simulink subsystem "HeatSubsystem"  (R2021a)
settings: Solver=VariableStepAuto  StartTime=0.0  StopTime=10.0  RelTol=1e-3
values from neighbouring files (symbols this model uses):
  dif = [1.0 1.0 1.0 1.0]    [InitialInputsGenerate.m]    (also in initializer.m = [1.0 1.0 1.0 10])
  get = [17.0 16.0 16.0 17.0]    [InitialInputsGenerate.m]    (also in initializer.m)
  x0 = [16.5 16.5 16.5 16.5]    [InitialInputsGenerate.m]    (also in initializer.m)
undefined symbols (not defined in the file or in its folder): h1, h2, h3, h4
settings Model: Creator=Kendra  LastModifiedBy=Kendra

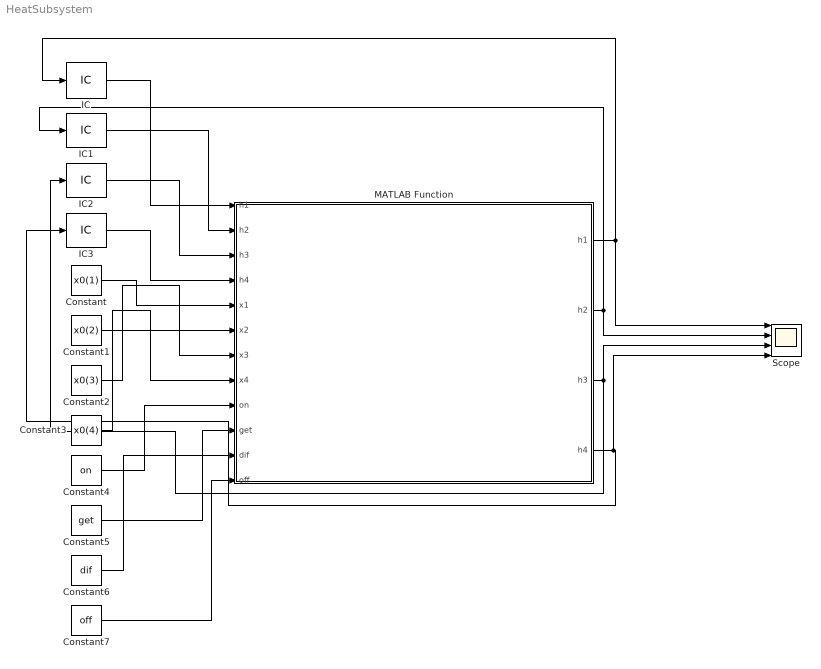
== system HeatSubsystem ==
  Constant : Constant  Value=x0(1)
  Constant1 : Constant  Value=x0(2)
  Constant2 : Constant  Value=x0(3)
  Constant3 : Constant  Value=x0(4)
  Constant4 : Constant  Value=on
  Constant5 : Constant  Value=get
  Constant6 : Constant  Value=dif
  Constant7 : Constant  Value=off
  IC : InitialCondition  Value=h1
  IC1 : InitialCondition  Value=h2
  IC2 : InitialCondition  Value=h3
  IC3 : InitialCondition  Value=h4
  MATLAB Function : MATLAB Function  TreatAsAtomicUnit=on
  Scope : Scope  NumInputPorts=4
  wires:
  IC3/1 -> MATLAB Function/4("h4 ")
  IC2/1 -> MATLAB Function/3("h3 ")
  IC1/1 -> MATLAB Function/2("h2 ")
  IC/1 -> MATLAB Function/1("h1 ")
  MATLAB Function/1(h1) -> IC/1, Scope/1
  MATLAB Function/2(h2) -> IC1/1, Scope/2
  MATLAB Function/3(h3) -> IC2/1, Scope/3
  MATLAB Function/4(h4) -> Scope/4, IC3/1
  Constant/1 -> MATLAB Function/5(x1)
  Constant1/1 -> MATLAB Function/6(x2)
  Constant2/1 -> MATLAB Function/7(x3)
  Constant3/1 -> MATLAB Function/8(x4)
  Constant4/1 -> MATLAB Function/9(on)
  Constant5/1 -> MATLAB Function/10(get)
  Constant6/1 -> MATLAB Function/11(dif)
  Constant7/1 -> MATLAB Function/12(off)

== matlab function HeatSubsystem/MATLAB Function ==
  data: h1 input; h1 output; h2 input; h3 input; h4 input; x1 input; x2 input; x3 input; x4 input; on input; get input; dif input; off input; h2 output; h3 output; h4 output
function [h1,h2,h3,h4] = SelectHeaters(h1,h2,h3,h4,x1,x2,x3,x4,on,get,dif,off)
x = [x1,x2,x3,x4];
h = [h1,h2,h3,h4];
hnew = h;
ind = find(h == 1);

biggestdiff = 0;
ind1 = 0;

for i = 1:1:4
    if x(i) <= on(i) && x(i) <= get(i) && x(i) < off(i) && x(ind(1)) - x(i) >= dif(i)
        curdiff = on(i)-x(i);
        if curdiff > biggestdiff
            biggestdiff = curdiff;
            ind1 = i;
        end
    end
end

hnew(ind(1)) = 0;
hnew(ind1) = 1;

biggestdiff = 0;
ind2 = 0;
for i = 1:1:4
    if x(i) <= on(i) && x(i) <= get(i) && x(i) < off(i) && x(ind(1)) - x(i) >= dif(i) && i ~= ind1
        curdiff = on(i)-x(i);
        if curdiff > biggestdiff
            biggestdiff = curdiff;
            ind2 = i;
        end
    end
end

hnew(ind(2)) = 0;
hnew(ind2) = 1;

h1 = hnew(1);
h2 = hnew(2);
h3 = hnew(3);
h4 = hnew(4);
